simulink model "teng4_VREP_panda_test_simulink"  (R2021a)
settings: Solver=FixedStepAuto  StartTime=0.0  StopTime=inf  RelTol=1e-3
values from neighbouring files (symbols this model uses):
  Q_des = [-0.9584 -0.9584 -0.9584 -0.9584 -0.9584 -0.9584 -0.9584 -0.9584 -0.9584 -0.9584 -0.9584 -0.9584 ... (143808 elements, 20544x7)]    [Q_des.mat]    (also in teng4_VREP_panda_test_traj_v1.m = Q'; teng4_VREP_panda_test_traj_v2.m = Q_des')
libraries: simulink x1
settings Model: Creator=Desktop-dds  LastModifiedBy=wan
settings SolverCC: AlgebraicLoopSolver=TrustRegion
settings DataIOCC: ReturnWorkspaceOutputs=off
settings DebuggingCC: SFMachineParentedDataDiag=warning  ArithmeticOperatorsInVariantConditions=warning
settings SFSimCC: CustomCodeUndefinedFunction=UseInterfaceOnly

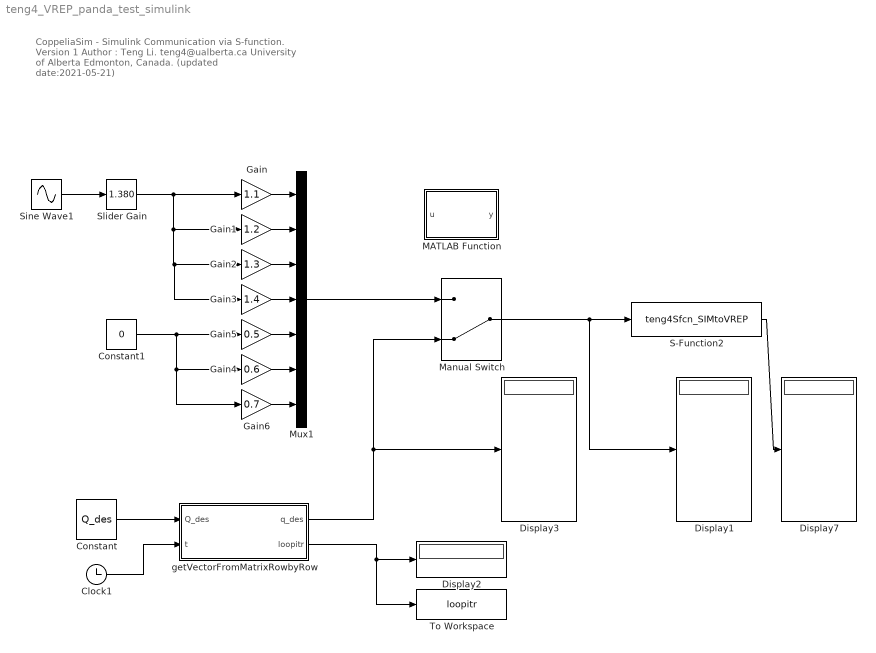
== system teng4_VREP_panda_test_simulink ==
  note: CoppeliaSim - Simulink Communication via S-function.
      | Version 1
      | Author : Teng Li.
      | teng4@ualberta.ca
      | University of Alberta
      | Edmonton, Canada.
      |
      | (updated date:2021-05-21)
  Clock1 : Clock
  Constant : Constant  Value=Q_des
  Constant1 : Constant  Value=0
  Display{1..3,7} (4 alike) : Display
  Gain : Gain  Gain=1.1
  Gain1 : Gain  Gain=1.2
  Gain2 : Gain  Gain=1.3
  Gain3 : Gain  Gain=1.4
  Gain4 : Gain  Gain=0.6
  Gain5 : Gain  Gain=0.5
  Gain6 : Gain  Gain=0.7
  MATLAB Function : MATLAB Function  TreatAsAtomicUnit=on
  Manual Switch : ManualSwitch  CurrentSetting=0
  Mux1 : Mux  Inputs=7
  S-Function2 : S-Function  FunctionName=teng4Sfcn_SIMtoVREP  SFunctionDeploymentMode=off  EnableBusSupport=off
  Sine Wave1 : Sin  SampleTime=0
  Slider Gain : simulink/Math Operations/Slider Gain  gain=1.380  low=0  high=3
  To Workspace : ToWorkspace  VariableName=loopitr  SaveFormat=Structure With Time  SampleTime=-1
  getVectorFromMatrixRowbyRow : MATLAB Function  TreatAsAtomicUnit=on
  wires:
  S-Function2/1 -> Display7/1
  Gain/1 -> Mux1/1
  Gain1/1 -> Mux1/2
  Gain2/1 -> Mux1/3
  Gain4/1 -> Mux1/6
  Gain6/1 -> Mux1/7
  Gain5/1 -> Mux1/5
  Gain3/1 -> Mux1/4
  Sine Wave1/1 -> Slider Gain/1
  Constant1/1 -> Gain6/1, Gain4/1, Gain5/1
  Mux1/1 -> Manual Switch/1
  Constant/1 -> getVectorFromMatrixRowbyRow/1(Q_des)
  Slider Gain/1 -> Gain3/1, Gain2/1, Gain1/1, Gain/1
  getVectorFromMatrixRowbyRow/2(loopitr) -> To Workspace/1, Display2/1
  Manual Switch/1 -> Display1/1, S-Function2/1
  Clock1/1 -> getVectorFromMatrixRowbyRow/2(t)
  getVectorFromMatrixRowbyRow/1(q_des) -> Display3/1, Manual Switch/2

== matlab function teng4_VREP_panda_test_simulink/getVectorFromMatrixRowbyRow ==
  data: Q_des input; q_des output; loopitr output; t input
function [q_des,loopitr] = fcn(Q_des,t)

Q_des=reshape(Q_des,[],7);
size_temp = size(Q_des);
size1=size_temp(1);


loop_i = round(t*1000)+1;
if loop_i>size1 %DONT exceed the length of the predefined matrix
    loop_i=size1;
end

q = Q_des(loop_i,1:7); %get one row from matrix Q_des.
q_des=reshape(q,[7,1]);

loopitr = loop_i; %for observation only.

== matlab function teng4_VREP_panda_test_simulink/MATLAB Function ==
  data: u input; y output
function y = fcn(u)

y = u;
